simulink model "combate"  (R2023b)
settings: Solver=FixedStepDiscrete  StartTime=0  StopTime=10  FixedStep=1  RelTol=1e-3
undefined symbols (not defined in the file): alpha_1, alpha_2, beta_1, beta_2, F0
settings Model: Creator=anruk  LastModifiedBy=anruk

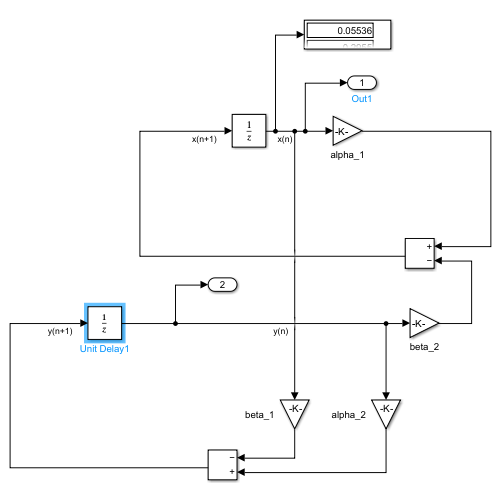
[thumbnail: Simulink's stored preview of the top-level diagram]
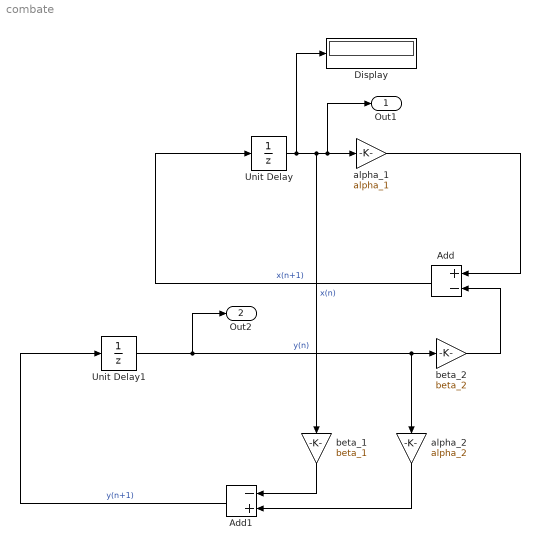
== system combate ==
  Add : Sum  Inputs=+-
  Add1 : Sum  Inputs=-+
  Display : Display
  Unit Delay : UnitDelay  InitialCondition=F0(1)  SampleTime=-1  HasFrameUpgradeWarning=on
  Unit Delay1 : UnitDelay  InitialCondition=F0(2)  SampleTime=-1  HasFrameUpgradeWarning=on
  alpha_1 : Gain  Gain=alpha_1
  alpha_2 : Gain  Gain=alpha_2
  beta_1 : Gain  Gain=beta_1
  beta_2 : Gain  Gain=beta_2
  Out1 : Outport
  Out2 : Outport  Port=2
  wires:
  Add/1 -> Unit Delay/1  "x(n+1)"
  Unit Delay/1 -> Display/1, Out1/1, alpha_1/1, beta_1/1  "x(n)"
  alpha_1/1 -> Add/1
  beta_2/1 -> Add/2
  Unit Delay1/1 -> Out2/1, beta_2/1, alpha_2/1  "y(n)"
  Add1/1 -> Unit Delay1/1  "y(n+1)"
  alpha_2/1 -> Add1/2
  beta_1/1 -> Add1/1
